simulink model "AMsb"  (Simulink 8.3)
settings: Solver=ode45  StartTime=0.0  StopTime=1  RelTol=1e-3
libraries: simulink x1, dsparch4 x1
settings Model: Creator=maalmasr  LastModifiedBy=maalmasr
settings SolverCC: ShapePreserveControl=EnableAll
settings DataIOCC: SignalLoggingName=sigsOut
settings OptimizationCC: ExpressionDepthLimit=2147483647
settings DebuggingCC: SaveWithParameterizedLinksMsg=none  UnderspecifiedInitializationDetection=Simplified  MergeDetectMultiDrivingBlocksExec=error  SignalResolutionControl=TryResolveAllWithWarning  SolverPrmCheckMsg=none  MultiTaskDSMMsg=warning  MultiTaskCondExecSysMsg=none  UnderSpecifiedDataTypeMsg=error
settings HardwareCC: TargetUnknown=on
settings ModelReferenceCC: EnableParallelModelReferenceBuilds=on
settings RTWCC: IncludeERTFirstTime=on

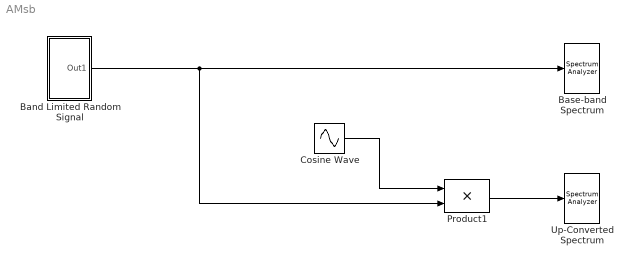
== system AMsb ==
  Band Limited Random Signal : Subsystem
  Base-band Spectrum : SpectrumAnalyzer  ScopeSpecification=DataTag1
  "Cosine Wave " : Sin  Frequency=3000*2*pi  SampleTime=1/16000
      settings: AttributesFormatString=Frequency = %<Frequency>
  Product1 : Product  SaturateOnIntegerOverflow=on  OutDataTypeStr=Inherit: Same as first input
  Up-Converted Spectrum : SpectrumAnalyzer  ScopeSpecification=DataTag2
  wires:
  Band Limited Random Signal/1(Out1) -> Product1/2, Base-band Spectrum/1
  "Cosine Wave "/1 -> Product1/1
  Product1/1 -> Up-Converted Spectrum/1

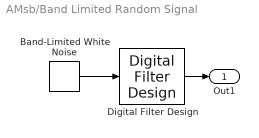
== system AMsb/Band Limited Random Signal ==
  Band-Limited White Noise : simulink/Sources/Band-Limited White Noise  Cov=10  Ts=1/16000  seed=[23341]
  Digital Filter Design : dsparch4/Digital Filter Design  mwdsp_browser_bugfix_var=off
  Out1 : Outport
  wires:
  Band-Limited White Noise/1 -> Digital Filter Design/1
  Digital Filter Design/1 -> Out1/1
